simulink model "simpleStateMachine"  (R2024b)
settings: Solver=VariableStepAuto  StartTime=0.0  StopTime=10.0  RelTol=1e-3
settings Model: Creator=optimus  LastModifiedBy=optimus

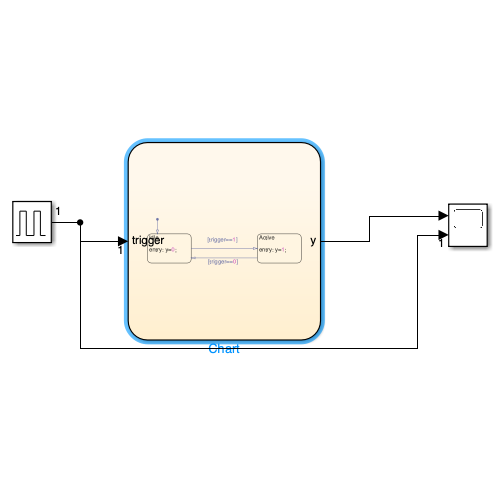
[thumbnail: Simulink's stored preview of the top-level diagram]
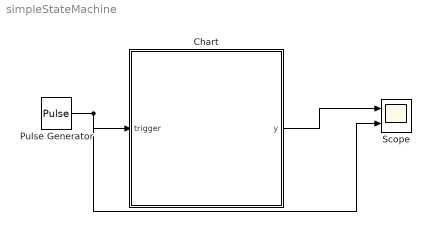
== system simpleStateMachine ==
  Chart : Stateflow chart  TreatAsAtomicUnit=on
  Pulse Generator : DiscretePulseGenerator  PulseType=Time based  PulseWidth=50
  Scope : Scope  NumInputPorts=2
  wires:
  Chart/1(y) -> Scope/1
  Pulse Generator/1 -> Scope/2, Chart/1(trigger)

== stateflow chart simpleStateMachine/Chart ==
  state Idle
    entry: y=0;
  state Active
    entry: y=1;
  (default) -> Idle
  Idle -> Active : [trigger==0]
  Active -> Idle : [trigger==1]
  data: trigger input double size=1; y output double size=1
